simulink model "ThrottleBody"  (R2024b)
settings: Solver=VariableStepAuto  StartTime=0.0  StopTime=10.0  RelTol=1e-3
model workspace (MAT data in the model file):
  c_damping = Simulink.Parameter
  c_damping.Value = 13
  c_damping.Complexity = 'real'
  c_damping.Dimensions = [1 1]
  c_damping.DataType = 'double'
  j_inertia = Simulink.Parameter
  j_inertia.Value = 0.2
  j_inertia.Complexity = 'real'
  j_inertia.Dimensions = [1 1]
  j_inertia.DataType = 'double'
  k_stiffness = Simulink.Parameter
  k_stiffness.Value = 1
  k_stiffness.Complexity = 'real'
  k_stiffness.Dimensions = [1 1]
  k_stiffness.DataType = 'double'
  kt = Simulink.Parameter
  kt.Value = 175
  kt.Complexity = 'real'
  kt.Dimensions = [1 1]
  kt.DataType = 'double'
  motordelay = Simulink.Parameter
  motordelay.Value = 0.01
  motordelay.Complexity = 'real'
  motordelay.Dimensions = [1 1]
  motordelay.DataType = 'double'
  openangle = Simulink.Parameter
  openangle.Value = 90
  openangle.Complexity = 'real'
  openangle.Dimensions = [1 1]
  openangle.DataType = 'double'
  restingangle = Simulink.Parameter
  restingangle.Value = 15
  restingangle.Complexity = 'real'
  restingangle.Dimensions = [1 1]
  restingangle.DataType = 'double'
settings Model: DataDictionary=SysMLArchModel_DD.sldd  ParameterArgumentNames=c_damping,j_inertia,k_stiffness,kt,motordelay,openangle,restingangle  Creator=ykamatan  LastModifiedBy=ykamatan

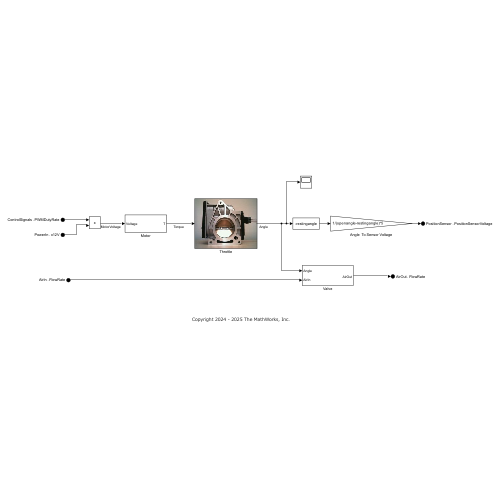
[thumbnail: Simulink's stored preview of the top-level diagram]
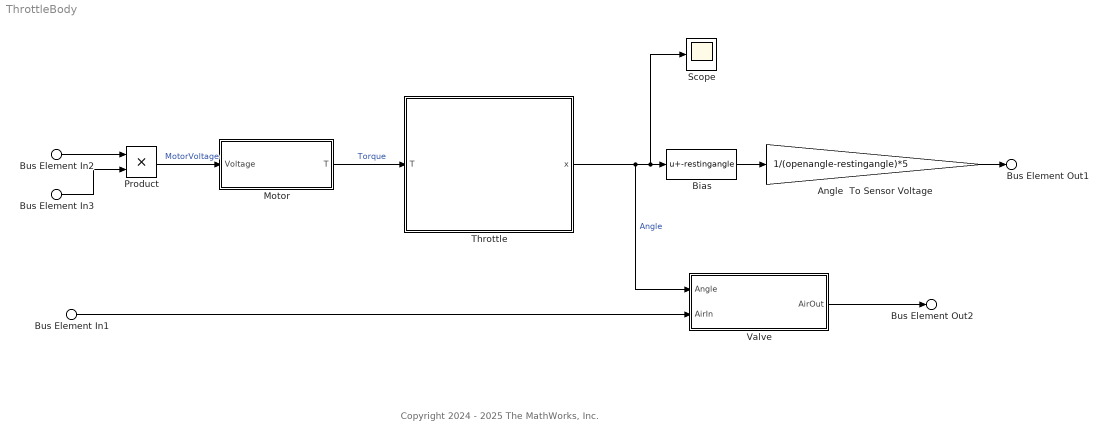
== system ThrottleBody ==
  note: Copyright 2024 - 2025 The MathWorks, Inc.
  Bus Element In1 : Inport  PortName=AirIn  Element=FlowRate
  Bus Element In2 : Inport  Port=2  PortName=ControlSignals  Element=PWMDutyRate
  Bus Element In3 : Inport  Port=3  PortName=PowerIn  Element=x12V
  Angle  To Sensor Voltage : Gain  Gain=1/(openangle-restingangle)*5
  Bias : Bias  Bias=-restingangle  SaturateOnIntegerOverflow=off
  Motor : Subsystem
  Product : Product
  Scope : Scope
  Throttle : Subsystem  mask{J=j_inertia, c=c_damping, k=k_stiffness, init=restingangle, open_val=openangle}
      mask prompts: J "Inertia:"; c "Damping:"; k "Stiffness:"; init "Resting Angle:"; open_val "Open Angle:"
      mask init:
      | throttle = imread('spe_engine_throttle.jpg');
      mask Display: image(throttle)
  Valve : Subsystem
  Bus Element Out1 : Outport  PortName=PositionSensor  Element=PositionSensorVoltage
  Bus Element Out2 : Outport  Port=2  PortName=AirOut  Element=FlowRate
  wires:
  Bus Element In3/1 -> Product/2
  Bus Element In2/1 -> Product/1
  Valve/1(AirOut) -> Bus Element Out2/1
  Product/1 -> Motor/1(Voltage)  "MotorVoltage"
  Throttle/1(x) -> Valve/1(Angle), Scope/1, Bias/1  "Angle"
  Motor/1(T) -> Throttle/1(T)  "Torque"
  Bus Element In1/1 -> Valve/2(AirIn)
  Bias/1 -> Angle  To Sensor Voltage/1
  Angle  To Sensor Voltage/1 -> Bus Element Out1/1

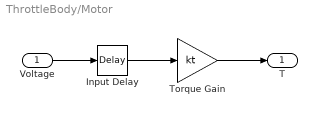
== system ThrottleBody/Motor ==
  Voltage : Inport
  Input Delay : TransportDelay  DelayTime=motordelay
  Torque Gain : Gain  Gain=kt  SaturateOnIntegerOverflow=on  OutDataTypeStr=Inherit: Same as input  ParamDataTypeStr=Inherit: Same as input
  T : Outport  VectorParamsAs1DForOutWhenUnconnected=off
  wires:
  Input Delay/1 -> Torque Gain/1
  Torque Gain/1 -> T/1
  Voltage/1 -> Input Delay/1

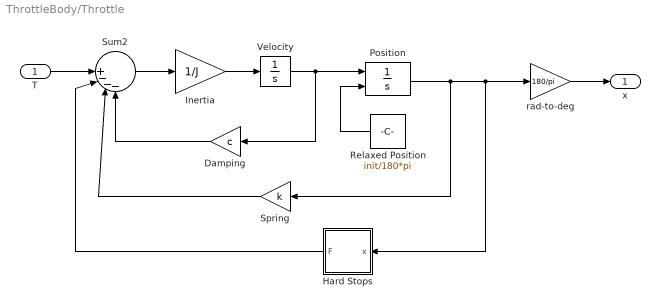
== system ThrottleBody/Throttle ==
  T : Inport
  Damping : Gain  Gain=c
  Hard Stops : Subsystem  mask{H=open_val/180*pi, K=2.86e5, L=init/180*pi}
      mask prompts: H "Upper Limit:"; K "Stiffness:"; L "Lower Limit:"
  Inertia : Gain  Gain=1/J  SaturateOnIntegerOverflow=on  OutDataTypeStr=Inherit: Same as input  ParamDataTypeStr=Inherit: Same as input
  Position : Integrator  InitialConditionSource=external
  Relaxed Position : Constant  Value=init/180*pi
  Spring : Gain  Gain=k
  Sum2 : Sum  Inputs=|||+---  InputSameDT=on  SaturateOnIntegerOverflow=on  OutDataTypeStr=Inherit: Same as first input
  Velocity : Integrator
  rad-to-deg : Gain  Gain=180/pi
  x : Outport  VectorParamsAs1DForOutWhenUnconnected=off
  wires:
  Spring/1 -> Sum2/3
  Damping/1 -> Sum2/4
  Position/1 -> Hard Stops/1(x), rad-to-deg/1, Spring/1
  Sum2/1 -> Inertia/1
  Inertia/1 -> Velocity/1
  Velocity/1 -> Position/1, Damping/1
  T/1 -> Sum2/1
  rad-to-deg/1 -> x/1
  Relaxed Position/1 -> Position/2
  Hard Stops/1(F) -> Sum2/2

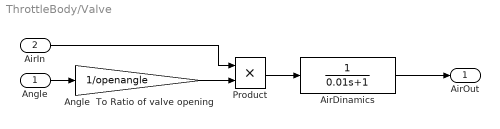
== system ThrottleBody/Valve ==
  Angle : Inport
  AirIn : Inport  Port=2
  AirDinamics : TransferFcn  Denominator=[0.01 1]
  Angle  To Ratio of valve opening : Gain  Gain=1/openangle
  Product : Product
  AirOut : Outport
  wires:
  Product/1 -> AirDinamics/1
  AirDinamics/1 -> AirOut/1
  AirIn/1 -> Product/1
  Angle  To Ratio of valve opening/1 -> Product/2
  Angle/1 -> Angle  To Ratio of valve opening/1

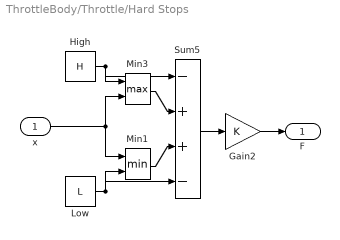
== system ThrottleBody/Throttle/Hard Stops ==
  x : Inport
  Gain2 : Gain  Gain=K  SaturateOnIntegerOverflow=on  OutDataTypeStr=Inherit: Same as input  ParamDataTypeStr=Inherit: Same as input
  High : Constant  Value=H
  Low : Constant  Value=L
  Min1 : MinMax  Inputs=2  InputSameDT=on  SaturateOnIntegerOverflow=on
  Min3 : MinMax  Function=max  Inputs=2  InputSameDT=on  SaturateOnIntegerOverflow=on
  Sum5 : Sum  Inputs=-+||+-  InputSameDT=on  SaturateOnIntegerOverflow=on  OutDataTypeStr=Inherit: Same as first input
  F : Outport  VectorParamsAs1DForOutWhenUnconnected=off
  wires:
  Min1/1 -> Sum5/3
  Min3/1 -> Sum5/2
  High/1 -> Min3/1, Sum5/1
  Low/1 -> Sum5/4, Min1/2
  Sum5/1 -> Gain2/1
  x/1 -> Min3/2, Min1/1
  Gain2/1 -> F/1
